simulink model "TuningCommandGeneratorTest"  (R2016b)
settings: Solver=FixedStepAuto  StartTime=0.0  StopTime=10.0  RelTol=1e-3  EnableMultiTasking=on
settings Model: Creator=march  LastModifiedBy=march
settings SolverCC: EnableConcurrentExecution=on
settings DataIOCC: SaveFormat=StructureWithTime
settings OptimizationCC: BlockReduction=off  OptimizeBlockIOStorage=off  BufferReuse=off  GlobalBufferReuse=off  ExpressionFolding=off  LocalBlockOutputs=off
settings HardwareCC: ProdBitPerPointer=32  ProdBitPerSizeT=32  ProdBitPerPtrDiffT=32  ProdLargestAtomicFloat=None  ProdWordSize=32  ProdLongLongMode=on  ProdHWDeviceType=Generic->32-bit x86 compatible
settings RTWCC: SystemTargetFile=slrt.tlc  TemplateMakefile=slrt_default_tmf  Description=Simulink Real-Time  RTWCompilerOptimization=on

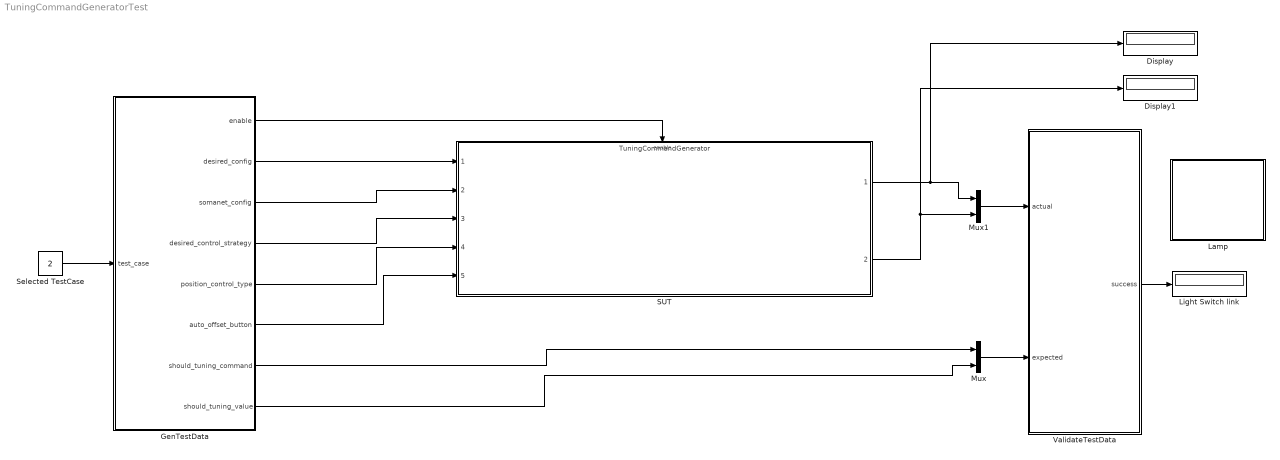
== system TuningCommandGeneratorTest ==
  Display : Display
  Display1 : Display
  GenTestData : MATLAB Function  TreatAsAtomicUnit=on
  Lamp : Subsystem  DialogController=hmiCreateDDGDialog  IsWebBlock=on  mask(MWDashboardBlock){webBlockId=5e27cf94-2efb-4dbd-a10c-411fdfea798e, webBlockType=lamp, ShowInLibBrowser=on, ShowInitialText=on, HMISrcModelName=TuningCommandGeneratorTest}
      mask prompts: webBlockType "WebBlock Type"; HMISrcModelName "Source Model"
      mask help: SimulinkHMI:dialogs:LampDialogDesc
      mask Help: helpview([docroot '/mapfiles/simulink.map'], 'hmi_lamp')
      mask Display:
      | if strcmp(get_param(bdroot(gcb),'BlockDiagramType'), 'library')
      |     image([(matlabroot) '/toolbox/simulink/hmi/icons/Lamp.png']);
      | end
  Light Switch link : Display
  Mux : Mux  Inputs=2
  Mux1 : Mux  Inputs=2
  SUT : ModelReference  ModelNameDialog=TuningCommandGenerator.slx  SimulationMode=Normal  ModelReferenceVersion=1.298  EnablePortName=Enable  EnablePortStatesWhenEnabling=held
  Selected TestCase : Constant  Value=2
  ValidateTestData : MATLAB Function  TreatAsAtomicUnit=on
  wires:
  Selected TestCase/1 -> GenTestData/1(test_case)
  GenTestData/2(desired_config) -> SUT/1
  GenTestData/3(somanet_config) -> SUT/2
  GenTestData/4(desired_control_strategy) -> SUT/3
  GenTestData/5(position_control_type) -> SUT/4
  GenTestData/6(auto_offset_button) -> SUT/5
  GenTestData/1(enable) -> SUT/Enable
  GenTestData/7(should_tuning_command) -> Mux/1
  GenTestData/8(should_tuning_value) -> Mux/2
  SUT/1 -> Display/1, Mux1/1
  SUT/2 -> Mux1/2, Display1/1
  ValidateTestData/1(success) -> Light Switch link/1
  Mux/1 -> ValidateTestData/2(expected)
  Mux1/1 -> ValidateTestData/1(actual)

== system TuningCommandGeneratorTest/Lamp ==

== matlab function TuningCommandGeneratorTest/ValidateTestData ==
  data: actual input; expected input; success output
function success = validate(actual,expected)
    success =0;
    assert(size(expected,1) == size(actual,1) && size(expected,2) == size(actual,2),'Size of input values do not match');
    
    
    for i=1:size(expected,1)
        assert(expected(i) == actual(i),'Test data does not match');
    end
    success =1;
end

== matlab function TuningCommandGeneratorTest/GenTestData ==
  data: enable output; test_case input; desired_config output; somanet_config output; desired_control_strategy output; position_control_type output; auto_offset_button output; should_tuning_command output; should_tuning_value output
function [enable,desired_config, somanet_config,desired_control_strategy,position_control_type,auto_offset_button,should_tuning_command,should_tuning_value] = TestDataGeneration(test_case)
%This function generates the testdata dependent on which test case is
%selected. It generates the test inputs as well as the expected outputs
%signaled with a preceeding should_
%To run one test case after another set testcase = -1

switch(test_case)
    case 1
        [enable,desired_config, somanet_config,desired_control_strategy,position_control_type,auto_offset_button,should_tuning_command,should_tuning_value] ...
            = testcase_kpp;
        return;
    otherwise
        [enable,desired_config, somanet_config,desired_control_strategy,position_control_type,auto_offset_button,should_tuning_command,should_tuning_value] ...
            = testcase_disabled;
end

end

function [enable,desired_config, somanet_config,desired_control_strategy,position_control_type,auto_offset_button,should_tuning_command,should_tuning_value] = testcase_disabled()
        %Default case for disabled subsystem
        desired_config = int32([900,21,-500000,+500000,4000,2000,500,0,700,10000,500,0,700,10000,0]);
        somanet_config = [900,21,-500000,+500000,4000,2000,500,0,700,10000,500,0,700,10000,0];
        desired_control_strategy = int8(1);
        position_control_type = int32(1);
        auto_offset_button = 0;
        enable = false;
        should_tuning_command = uint32(0);
        should_tuning_value = uint32(0);
end

function [enable,desired_config, somanet_config,desired_control_strategy,position_control_type,auto_offset_button,should_tuning_command,should_tuning_value] = testcase_kpp()
        %This case tests for a change in the p value of the position
        %controller
        desired_config = int32([900,21,-500000,+500000,4000,2000,500,0,700,10000,500,0,700,10000,0]);
        somanet_config = [900,21,-500000,+500000,4000,2000,300,0,700,10000,500,0,700,10000,0];
        desired_control_strategy = int8(1);
        position_control_type = int32(1);
        auto_offset_button = 0;
        enable = true;
        should_tuning_command = uint32(hex2dec('C0'));
        should_tuning_value = uint32(500);
end
